simulink model "simple_corr_audio_system_toolbox"  (Simulink 10.0)
settings: Solver=FixedStepDiscrete  StartTime=0.0  StopTime=1  RelTol=1e-3
PreLoadFcn:
  | load dspafxr;
libraries: dspsrcs4 x3, dspstat3 x2
settings Model: Creator=sv7  LastModifiedBy=water
settings SolverCC: PositivePriorityOrder=on
settings DataIOCC: SignalLoggingSaveFormat=ModelDataLogs  SaveOutput=off  SaveTime=off
settings OptimizationCC: DefaultParameterBehavior=Inlined  InlineInvariantSignals=on  ExpressionDepthLimit=2147483647  InitFltsAndDblsToZero=on  LifeSpan=1
settings DebuggingCC: SaveWithParameterizedLinksMsg=none  SignalResolutionControl=TryResolveAllWithWarning  SolverPrmCheckMsg=warning  MultiTaskDSMMsg=warning  MultiTaskCondExecSysMsg=none  FcnCallInpInsideContextMsg=warning  StateNameClashWarn=warning  SFExecutionAtInitializationDiag=warning
settings HardwareCC: ProdBitPerLong=40  ProdLargestAtomicInteger=Integer  ProdIntDivRoundTo=Zero  ProdEndianess=LittleEndian  ProdHWDeviceType=Texas Instruments->C6000  TargetBitPerLong=40  TargetLargestAtomicInteger=Integer  TargetIntDivRoundTo=Zero  TargetEndianess=LittleEndian  TargetHWDeviceType=TI C6000
settings RTWCC: Description=IDE Link ERT  SystemTargetFile=idelink_ert.tlc  GenerateMakefile=off  TemplateMakefile=none
settings TargetCC: CompOptLevelCompliant=off  ConcurrentExecutionCompliant=on  CombineOutputUpdateFcns=on  RemoveResetFunc=on  PreserveStateflowLocalDataDimensions=off  MATLABClassNameForMDSCustomization=linkfoundation.pjtgenerator.IdelinkCustomization  GRTInterface=off
settings CustomProperty: DataType=string
settings ConfigComp: CovExternalEMLEnable=off
settings TargetHardwareResources: Description=Target Hardware Resources Component
settings MATStruct: boardType=C6713DSK  isSimulator=[0.0]  enableHSRTDX=[0.0]  versionNumber=3.0  enableDSPBIOSTab=[0.0]  RTOS=DSP/BIOS  peripherals=[]  procName=CPU_1  boardName=C6713 DSK  realtimesupport=on  tag=ccslinktgtpref_ccsv5  deviceID=C6713  subFamily=671x  cpuClockRateMHz=[225.0]  codegenhookpoint=C6000  mvSwitch=-mv6710  numSections=[13.0]  numRTOS=[2.0]  defaultSysStackSize=[8192.0]  isBuiltIn=[1.0]  numBanks=[1.0]  numCacheLvl=[1.0]  isremovable=[0.0]  iscontentsfixed=[0.0]  name=IRAM  addr=[0.0]  size=[262144.0]  contents=Code & Data  space=Internal  createHeap=[0.0]  heapSize=[256.0]  defineLabel=[0.0]  heapLabel=segment_name  label=L2  timer=[]  timerprescaler=[]  description=C code  codeObjectMem=SDRAM  dataObjectMem=SDRAM  levelLabel=L2  cacheSize=64 kb  enable=off  schedulerType=Rate priority  schedulingMode=real-time  baseRatePriority=[7.0]  stackSize=[4096.0]  staticStackMemSegment=IRAM  dynamicStackMemSegment=SDRAM  errId=[]

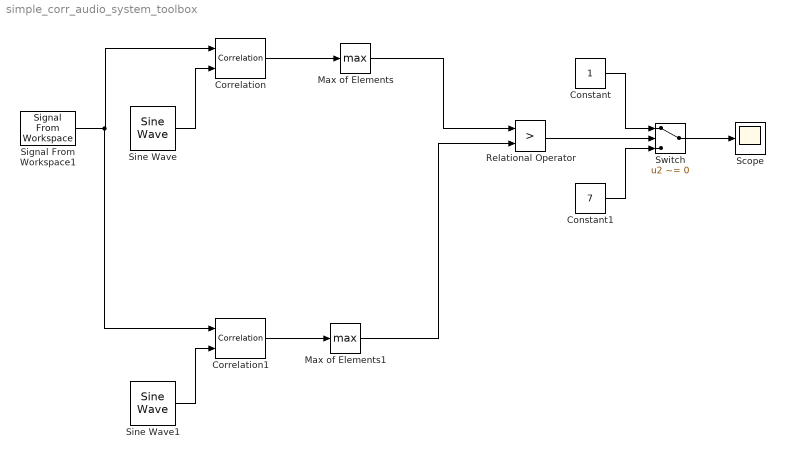
== system simple_corr_audio_system_toolbox ==
  Constant : Constant
  Constant1 : Constant  Value=7
  Correlation : dspstat3/Correlation  domain=Time  roundingMode=Floor  overflowMode=off  outputDataTypeStr=Inherit: Same as accumulator  outputMin=[]  outputMax=[]  outputLastDataTypeStr=Inherit: Same as accumulator
      settings: SourceProductName=DSP System Toolbox  SourceProductBaseCode=DS
  Correlation1 : dspstat3/Correlation  domain=Time  roundingMode=Floor  overflowMode=off  outputDataTypeStr=Inherit: Same as accumulator  outputMin=[]  outputMax=[]  outputLastDataTypeStr=Inherit: Same as accumulator
      settings: SourceProductName=DSP System Toolbox  SourceProductBaseCode=DS
  Max of Elements : MinMax  Function=max
  Max of Elements1 : MinMax  Function=max
  Relational Operator : RelationalOperator  Operator=>  OutDataTypeStr=boolean  RndMeth=Nearest
  Scope : Scope
  Signal From Workspace1 : dspsrcs4/Signal From Workspace  X=SinWave  Ts=1/8000  nsamps=40  OutputAfterFinalValue=Cyclic repetition  ignoreOrWarnInputAndFrameLengths=off  OutputFrames=on
  Sine Wave : dspsrcs4/Sine Wave  Amplitude=1  Frequency=697  Phase=0  SampleMode=Discrete  OutComplex=Real  CompMethod=Trigonometric fcn  TableSize=Speed  SampleTime=1/8000  SamplesPerFrame=40  ResetState=Restart at time zero  OutputFrames=off  dataType=double  wordLen=16  udDataType=sfix(16)  fracBitsMode=Best precision  numFracBits=15  OutDataTypeStr=double  LastOutDataTypeStr=double
  Sine Wave1 : dspsrcs4/Sine Wave  Amplitude=1  Frequency=1447  Phase=0  SampleMode=Discrete  OutComplex=Real  CompMethod=Trigonometric fcn  TableSize=Speed  SampleTime=1/8000  SamplesPerFrame=40  ResetState=Restart at time zero  OutputFrames=off  dataType=double  wordLen=16  udDataType=sfix(16)  fracBitsMode=Best precision  numFracBits=15  OutDataTypeStr=double  LastOutDataTypeStr=double
  Switch : Switch  Criteria=u2 ~= 0
  wires:
  Switch/1 -> Scope/1
  Relational Operator/1 -> Switch/2
  Constant1/1 -> Switch/3
  Constant/1 -> Switch/1
  Signal From Workspace1/1 -> Correlation1/1, Correlation/1
  Sine Wave/1 -> Correlation/2
  Sine Wave1/1 -> Correlation1/2
  Correlation/1 -> Max of Elements/1
  Max of Elements/1 -> Relational Operator/1
  Correlation1/1 -> Max of Elements1/1
  Max of Elements1/1 -> Relational Operator/2
